simulink model "Replay_Kalman_Filters"  (R2019a)
settings: Solver=ode1  StartTime=0.0  StopTime=PAR.finalTime  FixedStep=sampleTime  RelTol=1e-3
values from neighbouring files (symbols this model uses):
  filter = 3    [Validations_Script.m]
  Kalman_OP = Setup_Kalman_OP(Q, R)    [Validations_Script.m]
undefined symbols (not defined in the file or in its folder): DiscIntNeverNeededParam, Kalman_1_phi, Kalman_1_theta, Kalman_2_phi, Kalman_2_theta
settings Model: Creator=Gaming  LastModifiedBy=User

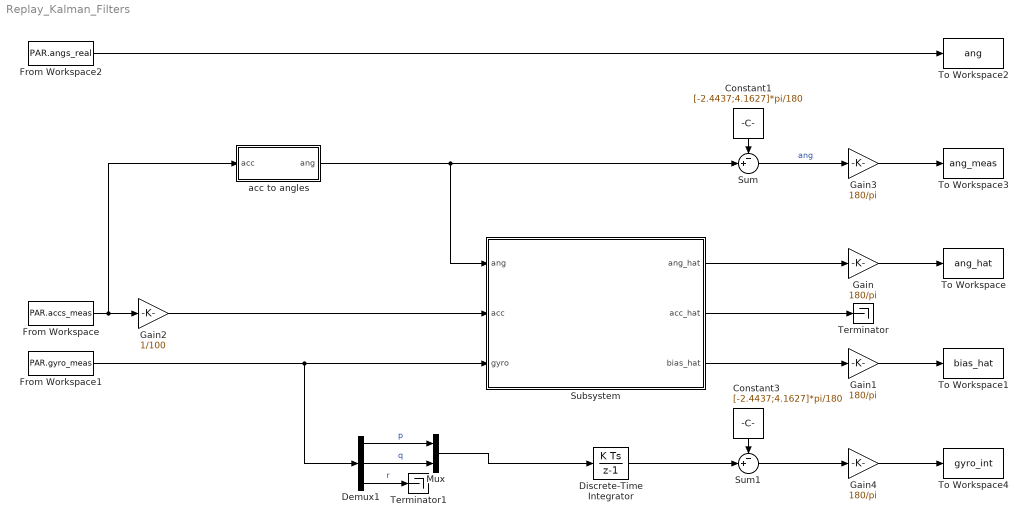
== system Replay_Kalman_Filters ==
  Constant1 : Constant  Value=[-2.4437;4.1627]*pi/180
  Constant3 : Constant  Value=[-2.4437;4.1627]*pi/180
  Demux1 : Demux  Outputs=3
  Discrete-Time Integrator : DiscreteIntegrator  SampleTime=-1  ICPrevOutput=DiscIntNeverNeededParam  ICPrevScaledInput=DiscIntNeverNeededParam
  From Workspace : FromWorkspace  VariableName=PAR.accs_meas  SampleTime=0
  From Workspace1 : FromWorkspace  VariableName=PAR.gyro_meas  SampleTime=0
  From Workspace2 : FromWorkspace  VariableName=PAR.angs_real  SampleTime=0
  Gain{,1,3..4} (4 alike) : Gain  Gain=180/pi
  Gain2 : Gain  Gain=1/100
  Mux : Mux  Inputs=2
  Subsystem : Subsystem
  Sum : Sum  Inputs=-+|
  Sum1 : Sum  Inputs=-+|
  Terminator : Terminator
  Terminator1 : Terminator
  To Workspace : ToWorkspace  VariableName=ang_hat  SaveFormat=Structure With Time  SampleTime=-1
  To Workspace1 : ToWorkspace  VariableName=bias_hat  SaveFormat=Structure With Time  SampleTime=-1
  To Workspace2 : ToWorkspace  VariableName=ang  SaveFormat=Structure With Time  SampleTime=-1
  To Workspace3 : ToWorkspace  VariableName=ang_meas  SaveFormat=Structure With Time  SampleTime=-1
  To Workspace4 : ToWorkspace  VariableName=gyro_int  SaveFormat=Structure With Time  SampleTime=-1
  acc to angles : MATLAB Function  TreatAsAtomicUnit=on
  wires:
  From Workspace/1 -> acc to angles/1(acc), Gain2/1
  Subsystem/1(ang_hat) -> Gain/1
  Gain/1 -> To Workspace/1
  Gain1/1 -> To Workspace1/1
  From Workspace2/1 -> To Workspace2/1
  Gain2/1 -> Subsystem/2(acc)
  From Workspace1/1 -> Demux1/1, Subsystem/3(gyro)
  Subsystem/2(acc_hat) -> Terminator/1
  Subsystem/3(bias_hat) -> Gain1/1
  Gain3/1 -> To Workspace3/1
  acc to angles/1(ang) -> Sum/2, Subsystem/1(ang)
  Constant1/1 -> Sum/1
  Sum/1 -> Gain3/1  "ang"
  Mux/1 -> Discrete-Time Integrator/1
  Discrete-Time Integrator/1 -> Sum1/2
  Sum1/1 -> Gain4/1
  Constant3/1 -> Sum1/1
  Demux1/3 -> Terminator1/1  "r"
  Demux1/1 -> Mux/1  "p"
  Demux1/2 -> Mux/2  "q"
  Gain4/1 -> To Workspace4/1

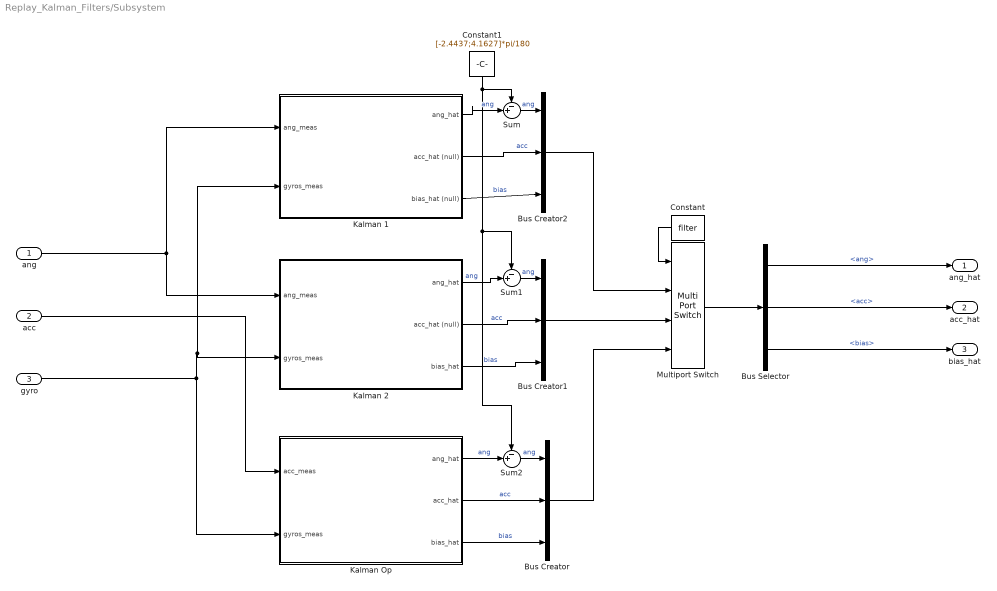
== system Replay_Kalman_Filters/Subsystem ==
  ang : Inport
  acc : Inport  Port=2
  gyro : Inport  Port=3
  Bus Creator : BusCreator  Inputs=3
  Bus Creator1 : BusCreator  Inputs=3
  Bus Creator2 : BusCreator  Inputs=3
  Bus Selector : BusSelector  OutputSignals=ang,acc,bias
  Constant : Constant  Value=filter
  Constant1 : Constant  Value=[-2.4437;4.1627]*pi/180
  Kalman 1 : Subsystem
  Kalman 2 : Subsystem
  Kalman Op : Subsystem
  Multiport Switch : MultiPortSwitch  AllowDiffInputSizes=on
  Sum : Sum  Inputs=-+|
  Sum1 : Sum  Inputs=-+|
  Sum2 : Sum  Inputs=-+|
  ang_hat : Outport
  acc_hat : Outport  Port=2
  bias_hat : Outport  Port=3
  wires:
  acc/1 -> Kalman Op/1(acc_meas)
  gyro/1 -> Kalman Op/2(gyros_meas), Kalman 1/2(gyros_meas), Kalman 2/2(gyros_meas)
  Multiport Switch/1 -> Bus Selector/1
  Bus Selector/3 -> bias_hat/1  "<bias>"
  Bus Selector/1 -> ang_hat/1  "<ang>"
  Bus Selector/2 -> acc_hat/1  "<acc>"
  Kalman Op/1(ang_hat) -> Sum2/2  "ang"
  Kalman Op/2(acc_hat) -> Bus Creator/2  "acc"
  Kalman Op/3(bias_hat) -> Bus Creator/3  "bias"
  Bus Creator/1 -> Multiport Switch/4
  Bus Creator1/1 -> Multiport Switch/3
  Bus Creator2/1 -> Multiport Switch/2
  Constant/1 -> Multiport Switch/1
  Kalman 2/1(ang_hat) -> Sum1/2  "ang"
  Kalman 2/2(acc_hat (null)) -> Bus Creator1/2  "acc"
  Kalman 2/3(bias_hat) -> Bus Creator1/3  "bias"
  Kalman 1/2(acc_hat (null)) -> Bus Creator2/2  "acc"
  Kalman 1/3(bias_hat (null)) -> Bus Creator2/3  "bias"
  Kalman 1/1(ang_hat) -> Sum/2  "ang"
  Sum/1 -> Bus Creator2/1  "ang"
  Constant1/1 -> Sum2/1, Sum1/1, Sum/1
  Sum2/1 -> Bus Creator/1  "ang"
  Sum1/1 -> Bus Creator1/1  "ang"
  ang/1 -> Kalman 2/1(ang_meas), Kalman 1/1(ang_meas)

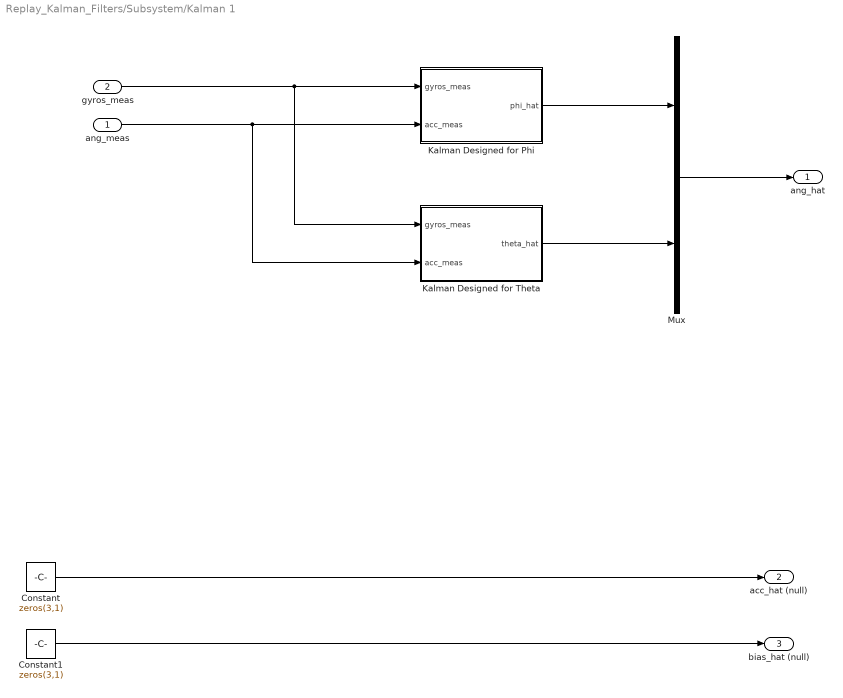
== system Replay_Kalman_Filters/Subsystem/Kalman 1 ==
  ang_meas : Inport
  gyros_meas : Inport  Port=2
  Constant : Constant  Value=zeros(3,1)
  Constant1 : Constant  Value=zeros(3,1)
  "Kalman Designed for Phi " : Subsystem
  Kalman Designed for Theta : Subsystem
  Mux : Mux  Inputs=2
  ang_hat : Outport  VectorParamsAs1DForOutWhenUnconnected=on
  acc_hat (null) : Outport  Port=2  VectorParamsAs1DForOutWhenUnconnected=on
  bias_hat (null) : Outport  Port=3  VectorParamsAs1DForOutWhenUnconnected=on
  wires:
  Constant/1 -> acc_hat (null)/1
  Constant1/1 -> bias_hat (null)/1
  gyros_meas/1 -> Kalman Designed for Theta/1(gyros_meas), "Kalman Designed for Phi "/1(gyros_meas)
  ang_meas/1 -> Kalman Designed for Theta/2(acc_meas), "Kalman Designed for Phi "/2(acc_meas)
  "Kalman Designed for Phi "/1(phi_hat) -> Mux/1
  Kalman Designed for Theta/1(theta_hat) -> Mux/2
  Mux/1 -> ang_hat/1

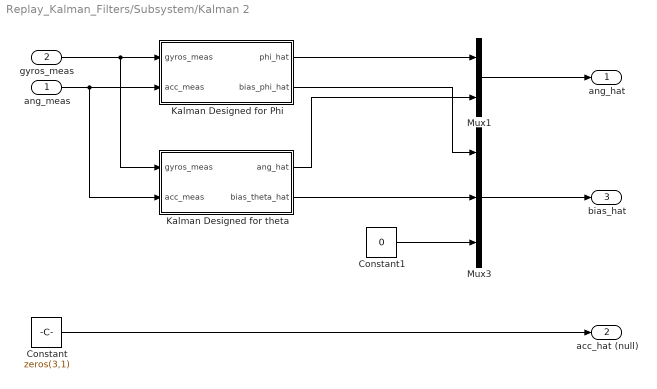
== system Replay_Kalman_Filters/Subsystem/Kalman 2 ==
  ang_meas : Inport
  gyros_meas : Inport  Port=2
  Constant : Constant  Value=zeros(3,1)
  Constant1 : Constant  Value=0
  Kalman Designed for Phi : Subsystem
  Kalman Designed for theta : Subsystem
  Mux1 : Mux  Inputs=2
  Mux3 : Mux  Inputs=3
  ang_hat : Outport  VectorParamsAs1DForOutWhenUnconnected=on
  acc_hat (null) : Outport  Port=2  VectorParamsAs1DForOutWhenUnconnected=on
  bias_hat : Outport  Port=3  VectorParamsAs1DForOutWhenUnconnected=on
  wires:
  Constant/1 -> acc_hat (null)/1
  gyros_meas/1 -> Kalman Designed for theta/1(gyros_meas), Kalman Designed for Phi/1(gyros_meas)
  ang_meas/1 -> Kalman Designed for theta/2(acc_meas), Kalman Designed for Phi/2(acc_meas)
  Mux3/1 -> bias_hat/1
  Constant1/1 -> Mux3/3
  Mux1/1 -> ang_hat/1
  Kalman Designed for Phi/1(phi_hat) -> Mux1/1
  Kalman Designed for theta/1(ang_hat) -> Mux1/2
  Kalman Designed for theta/2(bias_theta_hat) -> Mux3/2
  Kalman Designed for Phi/2(bias_phi_hat) -> Mux3/1

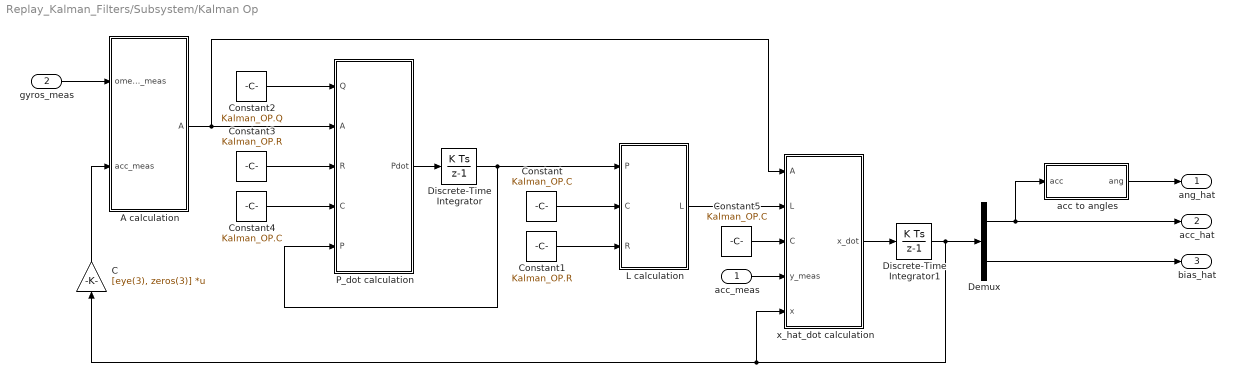
== system Replay_Kalman_Filters/Subsystem/Kalman Op ==
  acc_meas : Inport
  gyros_meas : Inport  Port=2
  A calculation : MATLAB Function  TreatAsAtomicUnit=on
  C : Gain  Gain=[eye(3), zeros(3)]  Multiplication=Matrix(K*u)
  Constant : Constant  Value=Kalman_OP.C
  Constant1 : Constant  Value=Kalman_OP.R
  Constant2 : Constant  Value=Kalman_OP.Q
  Constant3 : Constant  Value=Kalman_OP.R
  Constant4 : Constant  Value=Kalman_OP.C
  Constant5 : Constant  Value=Kalman_OP.C
  Demux : Demux  Outputs=2
  Discrete-Time Integrator : DiscreteIntegrator  InitialCondition=Kalman_OP.Q*10  SampleTime=-1  ICPrevOutput=DiscIntNeverNeededParam  ICPrevScaledInput=DiscIntNeverNeededParam
  Discrete-Time Integrator1 : DiscreteIntegrator  InitialCondition=zeros(6,1)  SampleTime=-1  ICPrevOutput=DiscIntNeverNeededParam  ICPrevScaledInput=DiscIntNeverNeededParam
  L calculation : MATLAB Function  TreatAsAtomicUnit=on
  P_dot calculation : MATLAB Function  TreatAsAtomicUnit=on
  acc to angles : MATLAB Function  TreatAsAtomicUnit=on
  x_hat_dot calculation : MATLAB Function  TreatAsAtomicUnit=on
  ang_hat : Outport
  acc_hat : Outport  Port=2
  bias_hat : Outport  Port=3
  wires:
  acc to angles/1(ang) -> ang_hat/1
  x_hat_dot calculation/1(x_dot) -> Discrete-Time Integrator1/1
  Discrete-Time Integrator1/1 -> Demux/1, x_hat_dot calculation/5(x), C/1
  L calculation/1(L) -> x_hat_dot calculation/2(L)
  P_dot calculation/1(Pdot) -> Discrete-Time Integrator/1
  Discrete-Time Integrator/1 -> P_dot calculation/5(P), L calculation/1(P)
  Constant/1 -> L calculation/2(C)
  Constant1/1 -> L calculation/3(R)
  Constant3/1 -> P_dot calculation/3(R)
  Constant2/1 -> P_dot calculation/1(Q)
  Demux/1 -> acc to angles/1(acc), acc_hat/1
  Demux/2 -> bias_hat/1
  acc_meas/1 -> x_hat_dot calculation/4(y_meas)
  gyros_meas/1 -> A calculation/1(omega_meas)
  A calculation/1(A) -> x_hat_dot calculation/1(A), P_dot calculation/2(A)
  Constant4/1 -> P_dot calculation/4(C)
  Constant5/1 -> x_hat_dot calculation/3(C)
  C/1 -> A calculation/2(acc_meas)

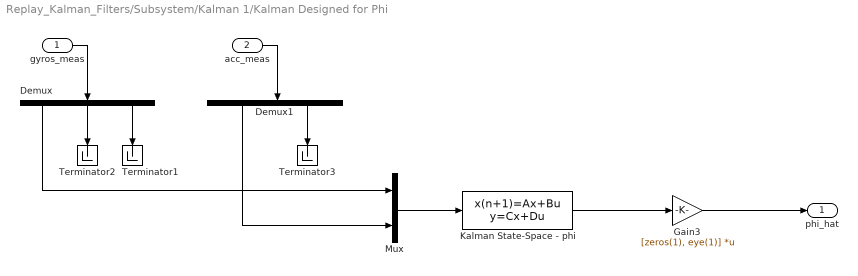
== system Replay_Kalman_Filters/Subsystem/Kalman 1/Kalman Designed for Phi  ==
  gyros_meas : Inport
  acc_meas : Inport  Port=2
  Demux : Demux  Outputs=3
  Demux1 : Demux  Outputs=2
  Gain3 : Gain  Gain=[zeros(1), eye(1)]  Multiplication=Matrix(K*u)
  Kalman State-Space - phi : DiscreteStateSpace  A=Kalman_1_phi.sys.A  B=Kalman_1_phi.sys.B  C=Kalman_1_phi.sys.C  D=Kalman_1_phi.sys.D  SampleTime=-1
  Mux : Mux  Inputs=2
  Terminator1 : Terminator
  Terminator2 : Terminator
  Terminator3 : Terminator
  phi_hat : Outport  VectorParamsAs1DForOutWhenUnconnected=on
  wires:
  Mux/1 -> Kalman State-Space - phi/1
  Kalman State-Space - phi/1 -> Gain3/1
  Demux/3 -> Terminator1/1
  Demux1/1 -> Mux/2
  Demux/1 -> Mux/1
  Gain3/1 -> phi_hat/1
  acc_meas/1 -> Demux1/1
  gyros_meas/1 -> Demux/1
  Demux/2 -> Terminator2/1
  Demux1/2 -> Terminator3/1

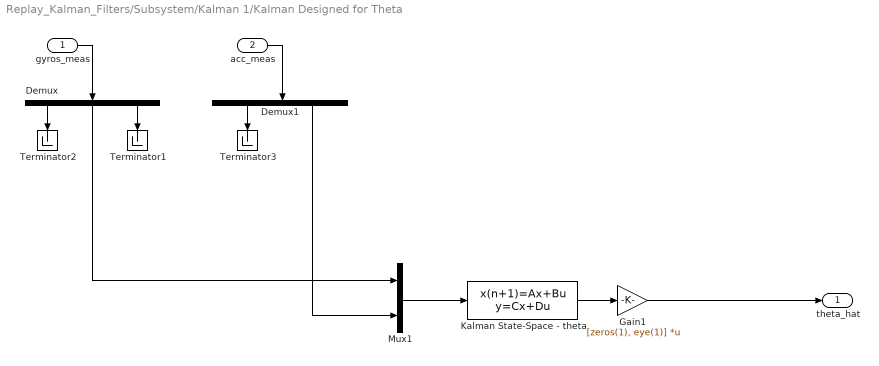
== system Replay_Kalman_Filters/Subsystem/Kalman 1/Kalman Designed for Theta ==
  gyros_meas : Inport
  acc_meas : Inport  Port=2
  Demux : Demux  Outputs=3
  Demux1 : Demux  Outputs=2
  Gain1 : Gain  Gain=[zeros(1), eye(1)]  Multiplication=Matrix(K*u)
  Kalman State-Space - theta : DiscreteStateSpace  A=Kalman_1_theta.sys.A  B=Kalman_1_theta.sys.B  C=Kalman_1_theta.sys.C  D=Kalman_1_theta.sys.D  SampleTime=-1
  Mux1 : Mux  Inputs=2
  Terminator1 : Terminator
  Terminator2 : Terminator
  Terminator3 : Terminator
  theta_hat : Outport  VectorParamsAs1DForOutWhenUnconnected=on
  wires:
  Demux/3 -> Terminator1/1
  Kalman State-Space - theta/1 -> Gain1/1
  Mux1/1 -> Kalman State-Space - theta/1
  Demux1/2 -> Mux1/2
  Gain1/1 -> theta_hat/1
  Demux/2 -> Mux1/1
  acc_meas/1 -> Demux1/1
  gyros_meas/1 -> Demux/1
  Demux/1 -> Terminator2/1
  Demux1/1 -> Terminator3/1

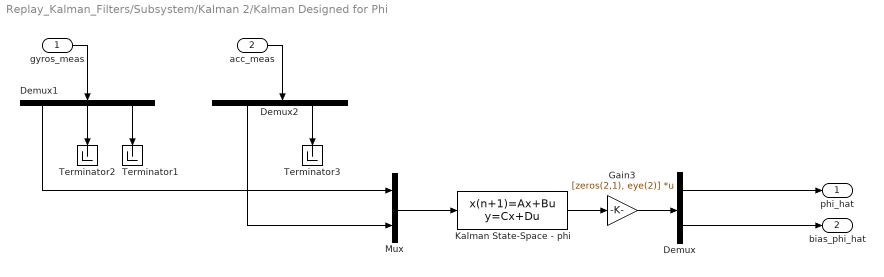
== system Replay_Kalman_Filters/Subsystem/Kalman 2/Kalman Designed for Phi ==
  gyros_meas : Inport
  acc_meas : Inport  Port=2
  Demux : Demux  Outputs=2
  Demux1 : Demux  Outputs=3
  Demux2 : Demux  Outputs=2
  Gain3 : Gain  Gain=[zeros(2,1), eye(2)]  Multiplication=Matrix(K*u)
  Kalman State-Space - phi : DiscreteStateSpace  A=Kalman_2_phi.sys.A  B=Kalman_2_phi.sys.B  C=Kalman_2_phi.sys.C  D=Kalman_2_phi.sys.D  SampleTime=-1
  Mux : Mux  Inputs=2
  Terminator1 : Terminator
  Terminator2 : Terminator
  Terminator3 : Terminator
  phi_hat : Outport  VectorParamsAs1DForOutWhenUnconnected=on
  bias_phi_hat : Outport  Port=2  VectorParamsAs1DForOutWhenUnconnected=on
  wires:
  Mux/1 -> Kalman State-Space - phi/1
  Demux1/1 -> Mux/1
  Demux2/1 -> Mux/2
  Gain3/1 -> Demux/1
  Demux/1 -> phi_hat/1
  Demux1/3 -> Terminator1/1
  acc_meas/1 -> Demux2/1
  Kalman State-Space - phi/1 -> Gain3/1
  gyros_meas/1 -> Demux1/1
  Demux/2 -> bias_phi_hat/1
  Demux1/2 -> Terminator2/1
  Demux2/2 -> Terminator3/1

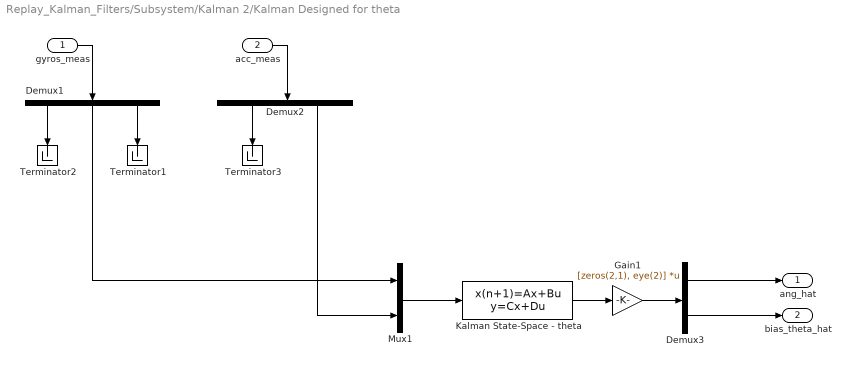
== system Replay_Kalman_Filters/Subsystem/Kalman 2/Kalman Designed for theta ==
  gyros_meas : Inport
  acc_meas : Inport  Port=2
  Demux1 : Demux  Outputs=3
  Demux2 : Demux  Outputs=2
  Demux3 : Demux  Outputs=2
  Gain1 : Gain  Gain=[zeros(2,1), eye(2)]  Multiplication=Matrix(K*u)
  Kalman State-Space - theta : DiscreteStateSpace  A=Kalman_2_theta.sys.A  B=Kalman_2_theta.sys.B  C=Kalman_2_theta.sys.C  D=Kalman_2_theta.sys.D  SampleTime=-1
  Mux1 : Mux  Inputs=2
  Terminator1 : Terminator
  Terminator2 : Terminator
  Terminator3 : Terminator
  ang_hat : Outport  VectorParamsAs1DForOutWhenUnconnected=on
  bias_theta_hat : Outport  Port=2  VectorParamsAs1DForOutWhenUnconnected=on
  wires:
  Demux1/2 -> Mux1/1
  Demux3/1 -> ang_hat/1
  Gain1/1 -> Demux3/1
  Demux2/2 -> Mux1/2
  Mux1/1 -> Kalman State-Space - theta/1
  Demux1/3 -> Terminator1/1
  acc_meas/1 -> Demux2/1
  Kalman State-Space - theta/1 -> Gain1/1
  gyros_meas/1 -> Demux1/1
  Demux3/2 -> bias_theta_hat/1
  Demux1/1 -> Terminator2/1
  Demux2/1 -> Terminator3/1

== matlab function Replay_Kalman_Filters/Subsystem/Kalman Op/A calculation ==
  data: omega_meas input; A output; acc_meas input
function A = fcn(omega_meas, acc_meas)

w = omega_meas;
a = acc_meas;

s_1 = [ 0   , -w(3) ,  w(2) ;...
        w(3),  0    , -w(1) ;...
       -w(2),  w(1) ,  0    ];
   
s_2 = [ 0   , -a(3) ,  a(2) ;...
        a(3),  0    , -a(1) ;...
       -a(2),  a(1) ,  0    ];
   
A = [-s_1, -s_2 ;...
     zeros(3,6) ];

== matlab function Replay_Kalman_Filters/Subsystem/Kalman Op/P_dot calculation ==
  data: Q input; A input; Pdot output; R input; C input; P input
function Pdot = fcn(Q, A, R, C, P)

Pdot = A*P + P*transpose(A) + Q - P*transpose(C)*inv(R)*C*P;

== matlab function Replay_Kalman_Filters/Subsystem/Kalman Op/acc to angles ==
  data: acc input; ang output
function ang = fcn(acc)

phi = -atan2(acc(2),-acc(3));

theta = atan2(acc(1),sqrt(acc(2)^2+acc(3)^2));

ang = [phi; theta];

== matlab function Replay_Kalman_Filters/Subsystem/Kalman Op/L calculation ==
  data: P input; L output; C input; R input
function L = fcn(P, C, R)

L = P*transpose(C)*inv(R);

== matlab function Replay_Kalman_Filters/Subsystem/Kalman Op/x_hat_dot calculation ==
  data: A input; x_dot output; L input; C input; y_meas input; x input
function x_dot = fcn(A,L,C,y_meas,x)

x_dot = A*x + L*(y_meas - C*x);

== matlab function Replay_Kalman_Filters/acc to angles ==
  data: acc input; ang output
function ang = fcn(acc)

phi = -atan2(acc(2),-acc(3));

theta = atan2(acc(1),sqrt(acc(2)^2+acc(3)^2));

ang = [phi; theta];
